simulink model "Definition_mf_2"  (R2020b)
settings: Solver=VariableStepAuto  StartTime=0.0  StopTime=8.5  RelTol=1e-3
values from neighbouring files (symbols this model uses):
  b = 0.0000313    (= 3.13e-05)    [parametre.m]
  d = 0.00000075    (= 7.5e-07)    [parametre.m]
  Ix = 0.0075    [parametre.m]
  Iy = 0.0075    [parametre.m]
  Iz = 0.013    [parametre.m]
  J = 0.00006    (= 6e-05)    [parametre.m]
  Jt = 0.0000604    (= 6.04e-05)    [parametre.m]
  k = 5.2*(10^(-3))    (= 0.0052)    [parametre.m]
  l = 0.23    [parametre.m]
  nu = 90    [parametre.m]
  r = 1/4    (= 0.25)    [parametre.m]
  to = ((R*Jt)/(k^2))    (= 1.34023668639)    [parametre.m]
libraries: pid_lib x3
settings Model: Creator=momen  LastModifiedBy=momen

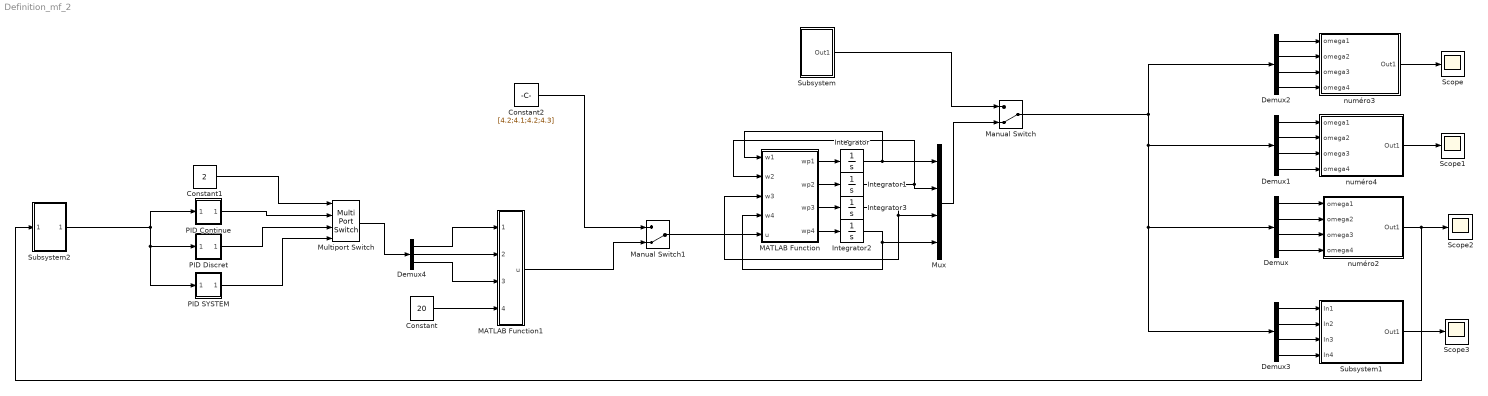
== system Definition_mf_2 ==
  Constant : Constant  Value=20
  Constant1 : Constant  Value=2
  Constant2 : Constant  Value=[4.2;4.1;4.2;4.3]
  Demux{,1..3} (4 alike) : Demux
  Demux4 : Demux  Outputs=3
  Integrator{,1..3} (4 alike) : Integrator
  MATLAB Function : MATLAB Function  TreatAsAtomicUnit=on
  MATLAB Function1 : MATLAB Function  TreatAsAtomicUnit=on
  Manual Switch : ManualSwitch  CurrentSetting=0
  Manual Switch1 : ManualSwitch  CurrentSetting=0
  Multiport Switch : MultiPortSwitch
  Mux : Mux
  PID Continue : Subsystem
  PID Discret : Subsystem
  PID SYSTEM : Subsystem
  Scope{,1..3} (4 alike) : Scope
  Subsystem : Subsystem
  Subsystem1 : Subsystem
  Subsystem2 : Subsystem
  numéro2 : Subsystem
  numéro3 : Subsystem
  numéro4 : Subsystem
  wires:
  numéro4/1(Out1) -> Scope1/1
  numéro2/1(Out1) -> Subsystem2/1(In1), Scope2/1
  Demux2/1 -> numéro3/1(omega1)
  Demux2/2 -> numéro3/2(omega2)
  Demux2/3 -> numéro3/3(omega3)
  Demux2/4 -> numéro3/4(omega4)
  Demux1/1 -> numéro4/1(omega1)
  Demux1/2 -> numéro4/2(omega2)
  Demux1/3 -> numéro4/3(omega3)
  Demux1/4 -> numéro4/4(omega4)
  Demux/4 -> numéro2/4(omega4)
  Demux/3 -> numéro2/3(omega3)
  Demux/2 -> numéro2/2(omega2)
  Demux/1 -> numéro2/1(omega1)
  Demux3/1 -> Subsystem1/1(In1)
  Demux3/2 -> Subsystem1/2(In2)
  Demux3/3 -> Subsystem1/3(In3)
  Demux3/4 -> Subsystem1/4(In4)
  Subsystem1/1(Out1) -> Scope3/1
  Constant2/1 -> Manual Switch1/1
  MATLAB Function/1(wp1) -> Integrator/1
  MATLAB Function/2(wp2) -> Integrator1/1
  MATLAB Function/3(wp3) -> Integrator3/1
  MATLAB Function/4(wp4) -> Integrator2/1
  Manual Switch/1 -> Demux3/1, Demux/1, Demux1/1, Demux2/1
  Subsystem/1(Out1) -> Manual Switch/1
  Integrator/1 -> MATLAB Function/1(w1), Mux/1
  Integrator1/1 -> Mux/2, MATLAB Function/2(w2)
  Integrator3/1 -> Mux/3, MATLAB Function/3(w3)
  Integrator2/1 -> Mux/4, MATLAB Function/4(w4)
  Mux/1 -> Manual Switch/2
  Manual Switch1/1 -> MATLAB Function/5(u)
  MATLAB Function1/1(u) -> Manual Switch1/2
  Constant/1 -> MATLAB Function1/4(v4)
  numéro3/1(Out1) -> Scope/1
  Subsystem2/1(Out1) -> PID SYSTEM/1(In1), PID Discret/1(In1), PID Continue/1(In1)
  PID Continue/1(Out1) -> Multiport Switch/2
  Demux4/1 -> MATLAB Function1/1(v1)
  Demux4/2 -> MATLAB Function1/2(v2)
  Demux4/3 -> MATLAB Function1/3(v3)
  PID Discret/1(Out1) -> Multiport Switch/3
  Multiport Switch/1 -> Demux4/1
  Constant1/1 -> Multiport Switch/1
  PID SYSTEM/1(Out1) -> Multiport Switch/4

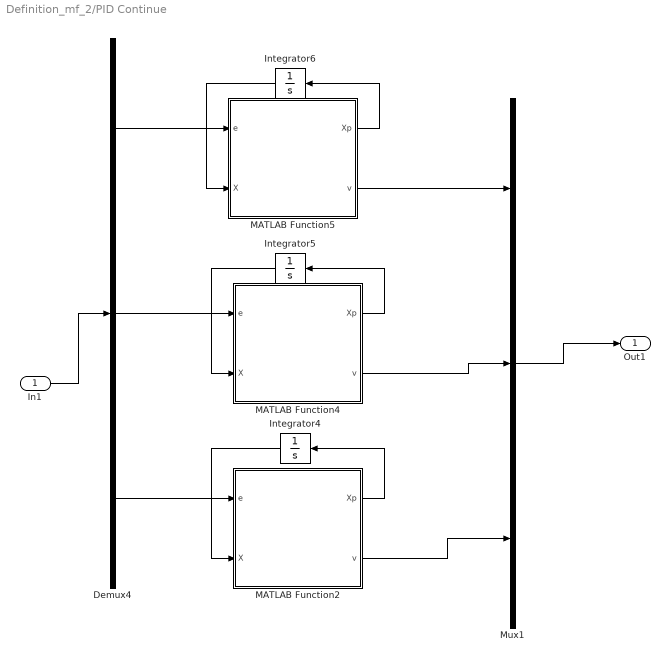
== system Definition_mf_2/PID Continue ==
  In1 : Inport
  Demux4 : Demux  Outputs=3
  Integrator4 : Integrator  InitialCondition=[0;0]
  Integrator5 : Integrator  InitialCondition=[0;0]
  Integrator6 : Integrator  InitialCondition=[0;0]
  MATLAB Function2 : MATLAB Function  TreatAsAtomicUnit=on
  MATLAB Function4 : MATLAB Function  TreatAsAtomicUnit=on
  MATLAB Function5 : MATLAB Function  TreatAsAtomicUnit=on
  Mux1 : Mux  Inputs=3
  Out1 : Outport
  wires:
  MATLAB Function5/1(Xp) -> Integrator6/1
  MATLAB Function2/1(Xp) -> Integrator4/1
  Demux4/1 -> MATLAB Function5/1(e)
  Integrator6/1 -> MATLAB Function5/2(X)
  Integrator5/1 -> MATLAB Function4/2(X)
  MATLAB Function5/2(v) -> Mux1/1
  MATLAB Function4/2(v) -> Mux1/2
  Demux4/2 -> MATLAB Function4/1(e)
  MATLAB Function4/1(Xp) -> Integrator5/1
  MATLAB Function2/2(v) -> Mux1/3
  Demux4/3 -> MATLAB Function2/1(e)
  Integrator4/1 -> MATLAB Function2/2(X)
  Mux1/1 -> Out1/1
  In1/1 -> Demux4/1

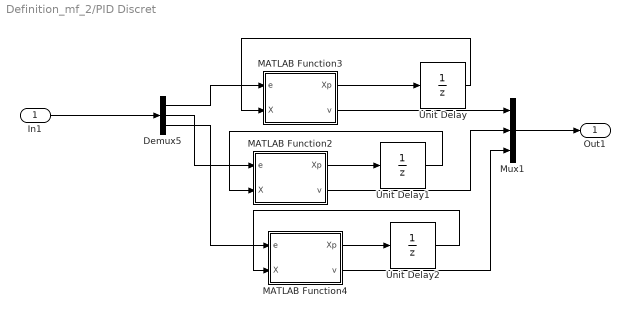
== system Definition_mf_2/PID Discret ==
  In1 : Inport
  Demux5 : Demux  Outputs=3
  MATLAB Function2 : MATLAB Function  TreatAsAtomicUnit=on
  MATLAB Function3 : MATLAB Function  TreatAsAtomicUnit=on
  MATLAB Function4 : MATLAB Function  TreatAsAtomicUnit=on
  Mux1 : Mux  Inputs=3
  Unit Delay : UnitDelay  InitialCondition=[0;0]  SampleTime=-1  HasFrameUpgradeWarning=on
  Unit Delay1 : UnitDelay  InitialCondition=[0;0]  SampleTime=-1  HasFrameUpgradeWarning=on
  Unit Delay2 : UnitDelay  InitialCondition=[0;0]  SampleTime=-1  HasFrameUpgradeWarning=on
  Out1 : Outport
  wires:
  MATLAB Function3/1(Xp) -> Unit Delay/1
  Unit Delay1/1 -> MATLAB Function2/2(X)
  MATLAB Function2/1(Xp) -> Unit Delay1/1
  Demux5/3 -> MATLAB Function4/1(e)
  MATLAB Function4/1(Xp) -> Unit Delay2/1
  MATLAB Function2/2(v) -> Mux1/2
  Unit Delay2/1 -> MATLAB Function4/2(X)
  Unit Delay/1 -> MATLAB Function3/2(X)
  Demux5/2 -> MATLAB Function2/1(e)
  MATLAB Function3/2(v) -> Mux1/1
  MATLAB Function4/2(v) -> Mux1/3
  Mux1/1 -> Out1/1
  Demux5/1 -> MATLAB Function3/1(e)
  In1/1 -> Demux5/1

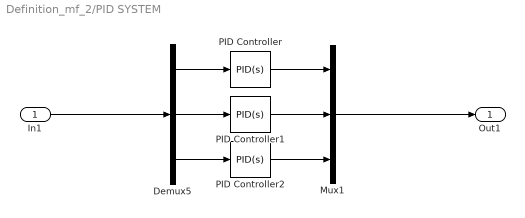
== system Definition_mf_2/PID SYSTEM ==
  In1 : Inport
  Demux5 : Demux  Outputs=3
  Mux1 : Mux  Inputs=3
  PID Controller : pid_lib/PID Controller  Controller=PID  Form=Parallel  TimeDomain=Continuous-time  UseExternalTs=off  SampleTime=-1  IntegratorMethod=Forward Euler  FilterMethod=Forward Euler  ControllerParametersSource=internal  P=0.9  I=0.3  D=0.2  UseFilter=on  N=100  TunerSelectOption=Transfer Function Based (PID Tuner App)  InitialConditionSource=internal  InitialConditionForIntegrator=0  InitialConditionForFilter=0  DifferentiatorICPrevScaledInput=0  ExternalReset=none  TrackingMode=off  Kt=1  LimitOutput=off  SatLimitsSource=internal  UpperSaturationLimit=inf  LowerSaturationLimit=-inf  LinearizeAsGain=on  AntiWindupMode=none  Kb=1  POutMin=[]  POutMax=[]  IOutMin=[]  IOutMax=[]  DOutMin=[]  DOutMax=[]  NOutMin=[]  NOutMax=[]  SumOutMin=[]  SumOutMax=[]  SaturationOutMin=[]  SaturationOutMax=[]  PParamMin=[]  PParamMax=[]  IParamMin=[]  IParamMax=[]  DParamMin=[]  DParamMax=[]  NParamMin=[]  NParamMax=[]  KbParamMin=[]  KbParamMax=[]  KtParamMin=[]  KtParamMax=[]  KbOutMin=[]  KbOutMax=[]  KtOutMin=[]  KtOutMax=[]  IntegratorOutMin=[]  IntegratorOutMax=[]  FilterOutMin=[]  FilterOutMax=[]  SumI1OutMin=[]  SumI1OutMax=[]  SumI2OutMin=[]  SumI2OutMax=[]  SumI3OutMin=[]  SumI3OutMax=[]  SumI4OutMin=[]  SumI4OutMax=[]  SumDOutMin=[]  SumDOutMax=[]  DifferentiatorOutMin=[]  DifferentiatorOutMax=[]  FilterDiffOutCoefMin=[]  FilterDiffOutCoefMax=[]  ReciprocalOutMin=[]  ReciprocalOutMax=[]  SumDenOutMin=[]  SumDenOutMax=[]  SumNumOutMin=[]  SumNumOutMax=[]  DivideOutMin=[]  DivideOutMax=[]  UdiffTsProdOutMin=[]  UdiffTsProdOutMax=[]  NTsProdOutMin=[]  NTsProdOutMax=[]  UintegralTsProdOutMin=[]  UintegralTsProdOutMax=[]  UngainTsProdOutMin=[]  UngainTsProdOutMax=[]  IntegratorContinuousStateAttributes=''  IntegratorStateMustResolveToSignalObject=off  IntegratorRTWStateStorageClass=Auto  FilterContinuousStateAttributes=''  FilterStateMustResolveToSignalObject=off  FilterRTWStateStorageClass=Auto  ParallelPVariant=InternalParameters  IdealPVariant=Disabled  IVariant=InternalParameters  DVariant=InternalParameters  IntegratorVariant=Continuous  SatVariant=Disabled  AWVariant=Passthrough  PCopyVariant=Disabled  TRVariant=Disabled  FdbkBlocksVariant=Forward  IdealPFdbkVariant=Disabled  SatFdbkVariant=Disabled  DerivativeFilterVariant=ContFilter  NVariant=InternalParameters  NCopyVariant=Disabled  FilterICVariant=InternalICsFilter  IntegratorICVariant=InternalICs  ExternalResetVariant=Disabled  TRSumVariant=Passthrough  SumFdbkVariant=Disabled  SumVariant=Sum_PID  TsampFilterVariant=InternalTs  TsampNgainVariant=Passthrough  TsampIntegralVariant=Passthrough  ExternalSaturationOutDataTypeStr=Inherit: Same as second input
  PID Controller1 : pid_lib/PID Controller  Controller=PID  Form=Parallel  TimeDomain=Continuous-time  UseExternalTs=off  SampleTime=-1  IntegratorMethod=Forward Euler  FilterMethod=Forward Euler  ControllerParametersSource=internal  P=0.9  I=0.3  D=0.2  UseFilter=on  N=100  TunerSelectOption=Transfer Function Based (PID Tuner App)  InitialConditionSource=internal  InitialConditionForIntegrator=0  InitialConditionForFilter=0  DifferentiatorICPrevScaledInput=0  ExternalReset=none  TrackingMode=off  Kt=1  LimitOutput=off  SatLimitsSource=internal  UpperSaturationLimit=inf  LowerSaturationLimit=-inf  LinearizeAsGain=on  AntiWindupMode=none  Kb=1  POutMin=[]  POutMax=[]  IOutMin=[]  IOutMax=[]  DOutMin=[]  DOutMax=[]  NOutMin=[]  NOutMax=[]  SumOutMin=[]  SumOutMax=[]  SaturationOutMin=[]  SaturationOutMax=[]  PParamMin=[]  PParamMax=[]  IParamMin=[]  IParamMax=[]  DParamMin=[]  DParamMax=[]  NParamMin=[]  NParamMax=[]  KbParamMin=[]  KbParamMax=[]  KtParamMin=[]  KtParamMax=[]  KbOutMin=[]  KbOutMax=[]  KtOutMin=[]  KtOutMax=[]  IntegratorOutMin=[]  IntegratorOutMax=[]  FilterOutMin=[]  FilterOutMax=[]  SumI1OutMin=[]  SumI1OutMax=[]  SumI2OutMin=[]  SumI2OutMax=[]  SumI3OutMin=[]  SumI3OutMax=[]  SumI4OutMin=[]  SumI4OutMax=[]  SumDOutMin=[]  SumDOutMax=[]  DifferentiatorOutMin=[]  DifferentiatorOutMax=[]  FilterDiffOutCoefMin=[]  FilterDiffOutCoefMax=[]  ReciprocalOutMin=[]  ReciprocalOutMax=[]  SumDenOutMin=[]  SumDenOutMax=[]  SumNumOutMin=[]  SumNumOutMax=[]  DivideOutMin=[]  DivideOutMax=[]  UdiffTsProdOutMin=[]  UdiffTsProdOutMax=[]  NTsProdOutMin=[]  NTsProdOutMax=[]  UintegralTsProdOutMin=[]  UintegralTsProdOutMax=[]  UngainTsProdOutMin=[]  UngainTsProdOutMax=[]  IntegratorContinuousStateAttributes=''  IntegratorStateMustResolveToSignalObject=off  IntegratorRTWStateStorageClass=Auto  FilterContinuousStateAttributes=''  FilterStateMustResolveToSignalObject=off  FilterRTWStateStorageClass=Auto  ParallelPVariant=InternalParameters  IdealPVariant=Disabled  IVariant=InternalParameters  DVariant=InternalParameters  IntegratorVariant=Continuous  SatVariant=Disabled  AWVariant=Passthrough  PCopyVariant=Disabled  TRVariant=Disabled  FdbkBlocksVariant=Forward  IdealPFdbkVariant=Disabled  SatFdbkVariant=Disabled  DerivativeFilterVariant=ContFilter  NVariant=InternalParameters  NCopyVariant=Disabled  FilterICVariant=InternalICsFilter  IntegratorICVariant=InternalICs  ExternalResetVariant=Disabled  TRSumVariant=Passthrough  SumFdbkVariant=Disabled  SumVariant=Sum_PID  TsampFilterVariant=InternalTs  TsampNgainVariant=Passthrough  TsampIntegralVariant=Passthrough  ExternalSaturationOutDataTypeStr=Inherit: Same as second input
  PID Controller2 : pid_lib/PID Controller  Controller=PID  Form=Parallel  TimeDomain=Continuous-time  UseExternalTs=off  SampleTime=-1  IntegratorMethod=Forward Euler  FilterMethod=Forward Euler  ControllerParametersSource=internal  P=0.06  I=0.3  D=0.02  UseFilter=on  N=100  TunerSelectOption=Transfer Function Based (PID Tuner App)  InitialConditionSource=internal  InitialConditionForIntegrator=0  InitialConditionForFilter=0  DifferentiatorICPrevScaledInput=0  ExternalReset=none  TrackingMode=off  Kt=1  LimitOutput=off  SatLimitsSource=internal  UpperSaturationLimit=inf  LowerSaturationLimit=-inf  LinearizeAsGain=on  AntiWindupMode=none  Kb=1  POutMin=[]  POutMax=[]  IOutMin=[]  IOutMax=[]  DOutMin=[]  DOutMax=[]  NOutMin=[]  NOutMax=[]  SumOutMin=[]  SumOutMax=[]  SaturationOutMin=[]  SaturationOutMax=[]  PParamMin=[]  PParamMax=[]  IParamMin=[]  IParamMax=[]  DParamMin=[]  DParamMax=[]  NParamMin=[]  NParamMax=[]  KbParamMin=[]  KbParamMax=[]  KtParamMin=[]  KtParamMax=[]  KbOutMin=[]  KbOutMax=[]  KtOutMin=[]  KtOutMax=[]  IntegratorOutMin=[]  IntegratorOutMax=[]  FilterOutMin=[]  FilterOutMax=[]  SumI1OutMin=[]  SumI1OutMax=[]  SumI2OutMin=[]  SumI2OutMax=[]  SumI3OutMin=[]  SumI3OutMax=[]  SumI4OutMin=[]  SumI4OutMax=[]  SumDOutMin=[]  SumDOutMax=[]  DifferentiatorOutMin=[]  DifferentiatorOutMax=[]  FilterDiffOutCoefMin=[]  FilterDiffOutCoefMax=[]  ReciprocalOutMin=[]  ReciprocalOutMax=[]  SumDenOutMin=[]  SumDenOutMax=[]  SumNumOutMin=[]  SumNumOutMax=[]  DivideOutMin=[]  DivideOutMax=[]  UdiffTsProdOutMin=[]  UdiffTsProdOutMax=[]  NTsProdOutMin=[]  NTsProdOutMax=[]  UintegralTsProdOutMin=[]  UintegralTsProdOutMax=[]  UngainTsProdOutMin=[]  UngainTsProdOutMax=[]  IntegratorContinuousStateAttributes=''  IntegratorStateMustResolveToSignalObject=off  IntegratorRTWStateStorageClass=Auto  FilterContinuousStateAttributes=''  FilterStateMustResolveToSignalObject=off  FilterRTWStateStorageClass=Auto  ParallelPVariant=InternalParameters  IdealPVariant=Disabled  IVariant=InternalParameters  DVariant=InternalParameters  IntegratorVariant=Continuous  SatVariant=Disabled  AWVariant=Passthrough  PCopyVariant=Disabled  TRVariant=Disabled  FdbkBlocksVariant=Forward  IdealPFdbkVariant=Disabled  SatFdbkVariant=Disabled  DerivativeFilterVariant=ContFilter  NVariant=InternalParameters  NCopyVariant=Disabled  FilterICVariant=InternalICsFilter  IntegratorICVariant=InternalICs  ExternalResetVariant=Disabled  TRSumVariant=Passthrough  SumFdbkVariant=Disabled  SumVariant=Sum_PID  TsampFilterVariant=InternalTs  TsampNgainVariant=Passthrough  TsampIntegralVariant=Passthrough  ExternalSaturationOutDataTypeStr=Inherit: Same as second input
  Out1 : Outport
  wires:
  In1/1 -> Demux5/1
  Demux5/3 -> PID Controller2/1
  Demux5/1 -> PID Controller/1
  Demux5/2 -> PID Controller1/1
  Mux1/1 -> Out1/1
  PID Controller/1 -> Mux1/1
  PID Controller1/1 -> Mux1/2
  PID Controller2/1 -> Mux1/3

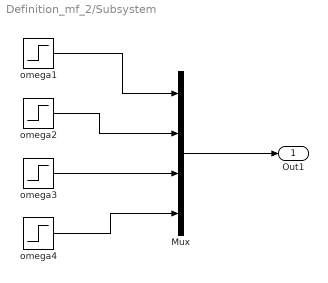
== system Definition_mf_2/Subsystem ==
  Mux : Mux
  omega{1..4} (4 alike) : Step  Time=2  After=150  SampleTime=0
  Out1 : Outport
  wires:
  omega3/1 -> Mux/3
  omega2/1 -> Mux/2
  omega1/1 -> Mux/1
  omega4/1 -> Mux/4
  Mux/1 -> Out1/1

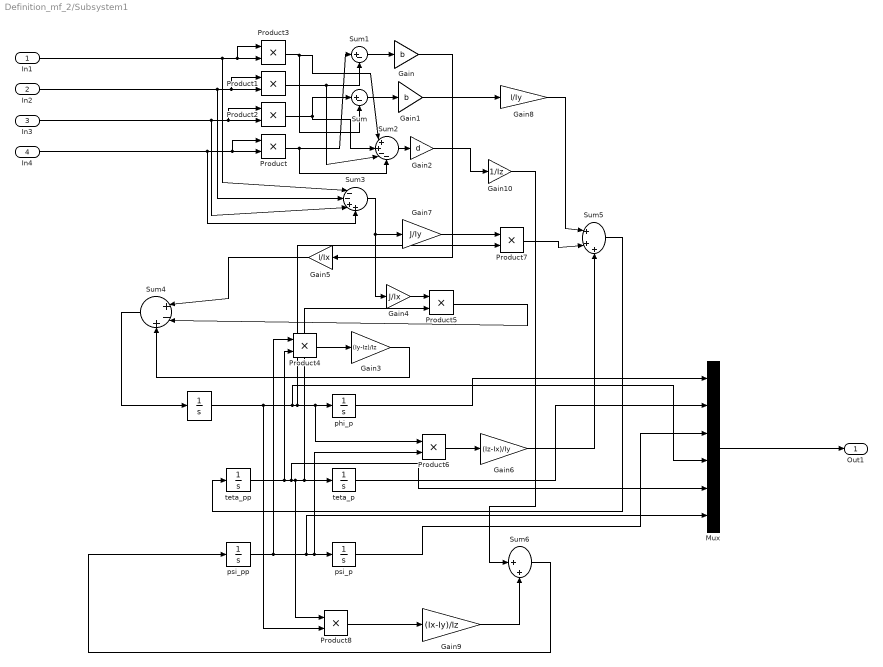
== system Definition_mf_2/Subsystem1 ==
  In1 : Inport
  In2 : Inport  Port=2
  In3 : Inport  Port=3
  In4 : Inport  Port=4
  " " : Integrator
  Gain : Gain  Gain=b
  Gain1 : Gain  Gain=b
  Gain10 : Gain  Gain=1/Iz
  Gain2 : Gain  Gain=d
  Gain3 : Gain  Gain=(Iy-Iz)/Iz
  Gain4 : Gain  Gain=J/Ix
  Gain5 : Gain  Gain=l/Ix
  Gain6 : Gain  Gain=(Iz-Ix)/Iy
  Gain7 : Gain  Gain=J/Iy
  Gain8 : Gain  Gain=l/Iy
  Gain9 : Gain  Gain=(Ix-Iy)/Iz
  Mux : Mux  Inputs=6
  Product{,1..8} (9 alike) : Product
  Sum : Sum  Inputs=|+-
  Sum1 : Sum  Inputs=|+-
  Sum2 : Sum  Inputs=|++--
  Sum3 : Sum  Inputs=|--++
  Sum4 : Sum  Inputs=|+-+
  Sum5 : Sum  Inputs=|+++
  Sum6 : Sum  Inputs=|++
  phi_p : Integrator
  psi_p : Integrator
  psi_pp : Integrator
  teta_p : Integrator
  teta_pp : Integrator
  Out1 : Outport
  wires:
  In2/1 -> Sum3/2, Product1/1, Product1/2
  Product8/1 -> Gain9/1
  Product5/1 -> Sum4/2
  Product2/1 -> Sum2/2, Sum/1
  Product1/1 -> Sum2/3, Sum1/2
  Product4/1 -> Gain3/1
  " "/1 -> Product8/2, Mux/4, Product7/2, Product6/1, phi_p/1
  Sum2/1 -> Gain2/1
  Product6/1 -> Gain6/1
  Gain6/1 -> Sum5/3
  In4/1 -> Sum3/4, Product/1, Product/2
  Sum1/1 -> Gain/1
  In1/1 -> Product3/2, Product3/1, Sum3/1
  teta_pp/1 -> Product4/2, Mux/5, Product8/1, teta_p/1, Product5/2
  Gain10/1 -> Sum6/1
  Sum3/1 -> Gain4/1, Gain7/1
  Product3/1 -> Sum2/1, Sum/2
  Gain8/1 -> Sum5/1
  psi_pp/1 -> Product4/1, Mux/6, Product6/2, psi_p/1
  Product/1 -> Sum2/4, Sum1/1
  Gain1/1 -> Gain8/1
  Gain9/1 -> Sum6/2
  Sum/1 -> Gain1/1
  Sum5/1 -> teta_pp/1
  Gain3/1 -> Sum4/3
  In3/1 -> Sum3/3, Product2/1, Product2/2
  Gain/1 -> Gain5/1
  Gain7/1 -> Product7/1
  Gain4/1 -> Product5/1
  Sum6/1 -> psi_pp/1
  teta_p/1 -> Mux/2
  phi_p/1 -> Mux/1
  Gain5/1 -> Sum4/1
  Sum4/1 -> " "/1
  Product7/1 -> Sum5/2
  psi_p/1 -> Mux/3
  Gain2/1 -> Gain10/1
  Mux/1 -> Out1/1

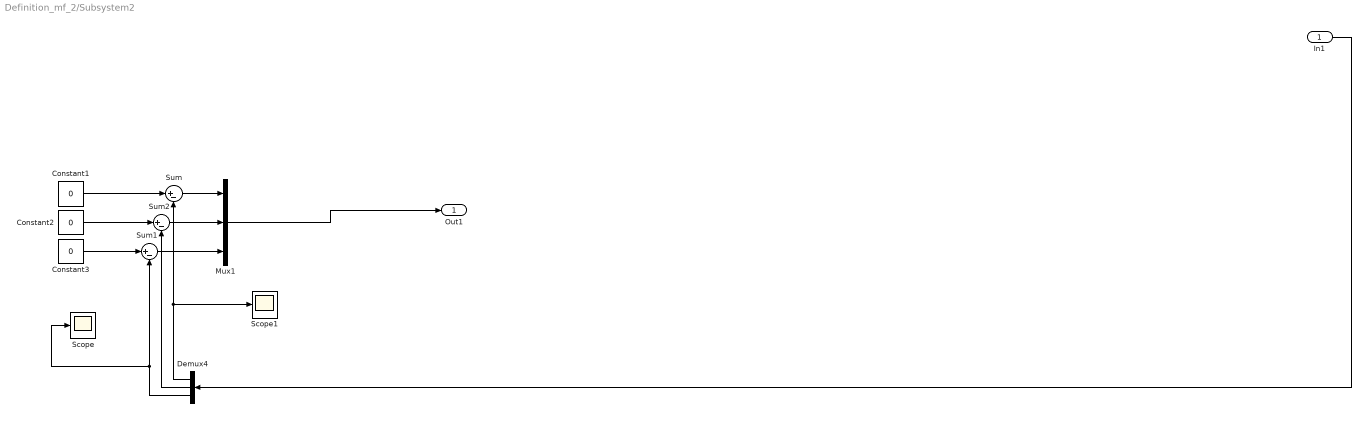
== system Definition_mf_2/Subsystem2 ==
  In1 : Inport
  Constant1 : Constant  Value=0
  Constant2 : Constant  Value=0
  Constant3 : Constant  Value=0
  Demux4 : Demux  Outputs=3
  Mux1 : Mux  Inputs=3
  Scope : Scope
  Scope1 : Scope
  Sum : Sum  Inputs=|+-
  Sum1 : Sum  Inputs=|+-
  Sum2 : Sum  Inputs=|+-
  Out1 : Outport
  wires:
  Demux4/1 -> Sum/2, Scope1/1
  Demux4/3 -> Scope/1, Sum1/2
  Sum1/1 -> Mux1/3
  Constant3/1 -> Sum1/1
  Demux4/2 -> Sum2/2
  Sum/1 -> Mux1/1
  Constant2/1 -> Sum2/1
  Constant1/1 -> Sum/1
  Sum2/1 -> Mux1/2
  Mux1/1 -> Out1/1
  In1/1 -> Demux4/1

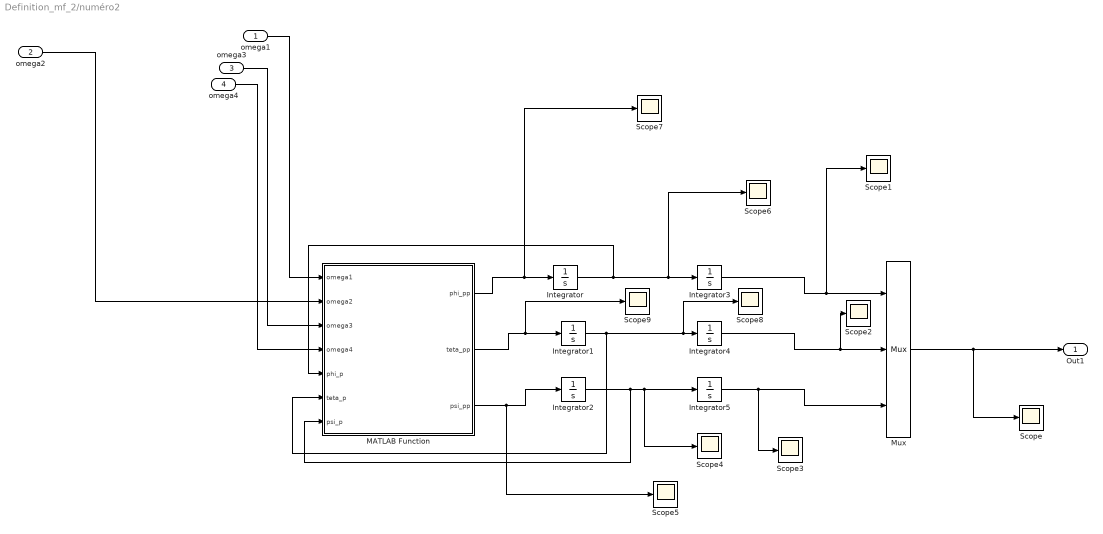
== system Definition_mf_2/numéro2 ==
  omega1 : Inport
  omega2 : Inport  Port=2
  omega3 : Inport  Port=3
  omega4 : Inport  Port=4
  Integrator : Integrator
  Integrator1 : Integrator
  Integrator2 : Integrator
  Integrator3 : Integrator  InitialCondition=pi/4
  Integrator4 : Integrator  InitialCondition=pi/4
  Integrator5 : Integrator  InitialCondition=pi/4
  MATLAB Function : MATLAB Function  TreatAsAtomicUnit=on
  Mux : Mux  Inputs=3
  Scope{,1..9} (10 alike) : Scope
  Out1 : Outport
  wires:
  Integrator3/1 -> Scope1/1, Mux/1
  MATLAB Function/2(teta_pp) -> Scope9/1, Integrator1/1
  Integrator1/1 -> MATLAB Function/6(teta_p), Scope8/1, Integrator4/1
  Integrator/1 -> MATLAB Function/5(phi_p), Scope6/1, Integrator3/1
  omega2/1 -> MATLAB Function/2(omega2)
  Integrator2/1 -> MATLAB Function/7(psi_p), Scope4/1, Integrator5/1
  Integrator4/1 -> Scope2/1, Mux/2
  MATLAB Function/1(phi_pp) -> Scope7/1, Integrator/1
  MATLAB Function/3(psi_pp) -> Scope5/1, Integrator2/1
  omega4/1 -> MATLAB Function/4(omega4)
  omega3/1 -> MATLAB Function/3(omega3)
  omega1/1 -> MATLAB Function/1(omega1)
  Mux/1 -> Scope/1, Out1/1
  Integrator5/1 -> Scope3/1, Mux/3

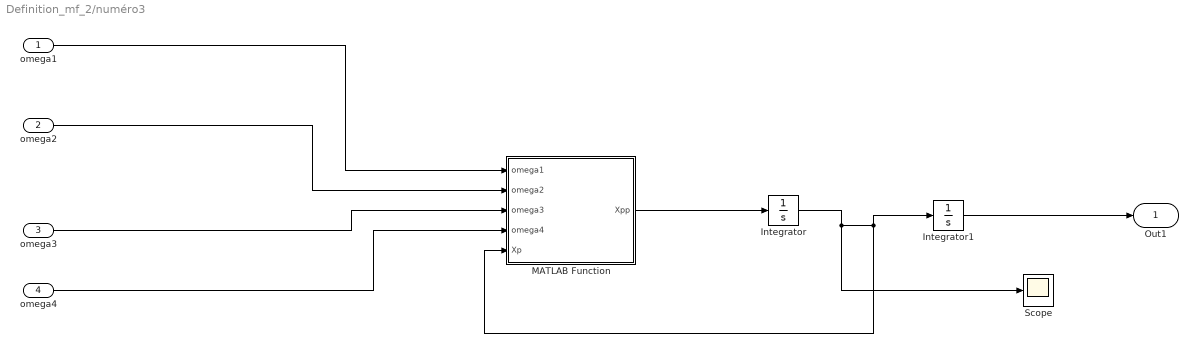
== system Definition_mf_2/numéro3 ==
  omega1 : Inport
  omega2 : Inport  Port=2
  omega3 : Inport  Port=3
  omega4 : Inport  Port=4
  Integrator : Integrator  InitialCondition=[0;0;0]
  Integrator1 : Integrator  InitialCondition=[0;0;0]
  MATLAB Function : MATLAB Function  TreatAsAtomicUnit=on
  Scope : Scope
  Out1 : Outport
  wires:
  MATLAB Function/1(Xpp) -> Integrator/1
  omega1/1 -> MATLAB Function/1(omega1)
  omega3/1 -> MATLAB Function/3(omega3)
  omega2/1 -> MATLAB Function/2(omega2)
  Integrator1/1 -> Out1/1
  omega4/1 -> MATLAB Function/4(omega4)
  Integrator/1 -> Scope/1, Integrator1/1, MATLAB Function/5(Xp)

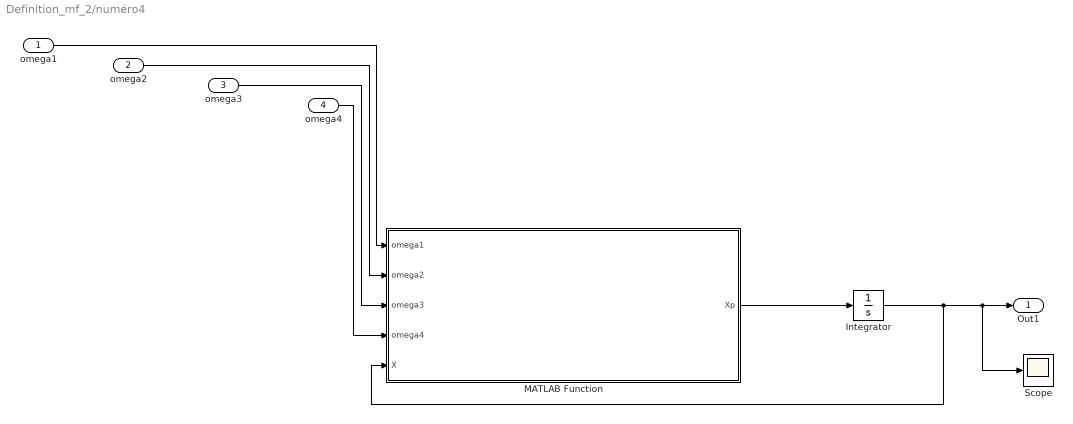
== system Definition_mf_2/numéro4 ==
  omega1 : Inport
  omega2 : Inport  Port=2
  omega3 : Inport  Port=3
  omega4 : Inport  Port=4
  Integrator : Integrator  InitialCondition=[0.785;0.785;0.785;0;0;0]
  MATLAB Function : MATLAB Function  TreatAsAtomicUnit=on
  Scope : Scope
  Out1 : Outport
  wires:
  Integrator/1 -> Scope/1, Out1/1, MATLAB Function/5(X)
  omega4/1 -> MATLAB Function/4(omega4)
  omega1/1 -> MATLAB Function/1(omega1)
  MATLAB Function/1(Xp) -> Integrator/1
  omega3/1 -> MATLAB Function/3(omega3)
  omega2/1 -> MATLAB Function/2(omega2)

== matlab function Definition_mf_2/MATLAB Function1 ==
  data: v1 input; u output; v2 input; v3 input; v4 input
function u = T(v1,v2,v3,v4)
u=[0;0;0;0];
u(1)=(-0.5*v2 -0.25*v3 + 0.25*v4 );
u(2)=(-0.5*v1 +0.25*v3 + 0.25*v4 );
u(3)=( 0.5*v2 -0.25*v3 + 0.25*v4 );
u(4)=( 0.5*v1 +0.25*v3 + 0.25*v4 );

== matlab function Definition_mf_2/PID Continue/MATLAB Function2 ==
  data: e input; Xp output; X input; v output
function [Xp,v]= fcn(e,X)
Kp=0.8
Ki=0
Kd=0.5
N= 100
Xp=[0;0];
Xp(1) = e;
Xp(2) = N*(Kd*e-X(2));
Xp=[Xp(1);Xp(2)];
v = Kp*e+Ki*X(1)+Xp(2);

== matlab function Definition_mf_2/PID Discret/MATLAB Function3 ==
  data: e input; Xp output; X input; v output; Te parameter
function [Xp,v]= fcn(e,X,Te)
Kp=0.8
Ki=0
Kd=0.4
N= 100
Xp=[0;0];
Xp(1) = X(1) + Te*e;
Xp(2) = X(2) +Te*N*(Kd*e-X(2));
Xp=[Xp(1);Xp(2)];
v = Kp*e+Ki*X(1)+N*(Kd*e-X(2));

== matlab function Definition_mf_2/PID Continue/MATLAB Function4 ==
  data: e input; Xp output; X input; v output
function [Xp,v]= fcn(e,X)
Kp=0.8
Ki=0
Kd=0.5
N= 100
Xp=[0;0];
Xp(1) = e;
Xp(2) = N*(Kd*e-X(2));
Xp=[Xp(1);Xp(2)];
v = Kp*e+Ki*X(1)+Xp(2);

== matlab function Definition_mf_2/PID Continue/MATLAB Function5 ==
  data: e input; Xp output; X input; v output
function [Xp,v]= fcn(e,X)
Kp=0.8
Ki=0
Kd=0.5
N= 100
Xp=[0;0];
Xp(1) = e;
Xp(2) = N*(Kd*e-X(2));
Xp=[Xp(1);Xp(2)];
v = Kp*e+Ki*X(1)+Xp(2);

== matlab function Definition_mf_2/PID Discret/MATLAB Function2 ==
  data: e input; Xp output; X input; v output; Te parameter
function [Xp,v]= fcn(e,X,Te)
Kp=0.8
Ki=0
Kd=0.4
N= 100
Xp=[0;0];
Xp(1) = X(1) + Te*e;
Xp(2) = X(2) +Te*N*(Kd*e-X(2));
Xp=[Xp(1);Xp(2)];
v = Kp*e+Ki*X(1)+N*(Kd*e-X(2));

== matlab function Definition_mf_2/PID Discret/MATLAB Function4 ==
  data: e input; Xp output; X input; v output; Te parameter
function [Xp,v]= fcn(e,X,Te)
Kp=0.8
Ki=0
Kd=0.5
N= 100
Xp=[0;0];
Xp(1) = X(1) + Te*e;
Xp(2) = X(2) +Te*N*(Kd*e-X(2));
Xp=[Xp(1);Xp(2)];
v = Kp*e+Ki*X(1)+N*(Kd*e-X(2));

== matlab function Definition_mf_2/numéro4/MATLAB Function ==
  data: omega1 input; Xp output; omega2 input; omega3 input; omega4 input; X input; Ix parameter; Iy parameter; Iz parameter; J parameter; b parameter; d parameter; l parameter
function Xp = n4(omega1,omega2,omega3,omega4,X,Ix, Iy, Iz, J, b, d, l)
Xp = [0;0;0;0;0;0];
U1 = 0;
U2 = 0;
U3 = 0;
omega =0;
U1 = b*((omega4^2)-(omega2^2));
U2 = b*(omega3^2-omega1^2);
U3 = d*(-omega1^2-omega3^2+omega2^2+omega4^2);
omega = omega2+omega4-omega1-omega3;
Xp(1) = X(4);
Xp(2) = X(5);
Xp(3) = X(6);
Xp(4) = X(5)*X(6)*((Iy-Iz)/Ix)-(J/Ix)*X(5)*omega +(l/Ix)*U1;
Xp(5) = X(4)*X(6)*((Iz-Ix)/Iy)+(J/Iy)*X(4)*omega +(l/Ix)*U2;
Xp(6) = X(4)*X(5)*((Ix-Iy)/Iz)+(1/Iz)*U3;
Xp = [Xp(1);Xp(2);Xp(3);Xp(4);Xp(5);Xp(6)];

== matlab function Definition_mf_2/numéro3/MATLAB Function ==
  data: omega1 input; Xpp output; omega2 input; omega3 input; omega4 input; Xp input; Ix parameter; Iy parameter; Iz parameter; J parameter; b parameter; d parameter; l parameter
function Xpp = n3(omega1,omega2,omega3,omega4,Xp,Ix, Iy, Iz, J,b, d,l)
Xpp = [0; 0; 0];
U1 = 0;
U2 = 0;
U3 = 0;
omega = 0;
U1 = b*((omega4^2)-(omega2^2));
U2 = b*(omega3^2-omega1^2);
U3 = d*(omega1^2+omega3^2-omega2^2-omega4^2);
omega = omega2+omega4-omega1-omega3;
Xpp(1) = Xp(2)*Xp(3)*((Iy-Iz)/Ix)-(J/Ix)*Xp(2)*omega +(l/Ix)*U1;
Xpp(2) = Xp(1)*Xp(3)*((Iz-Ix)/Iy)+(J/Iy)*Xp(1)*omega +(l/Ix)*U2;
Xpp(3) = Xp(1)*Xp(2)*((Ix-Iy)/Iz)+(1/Iz)*U3;
Xpp = [Xpp(1); Xpp(2);Xpp(3)];

== matlab function Definition_mf_2/numéro2/MATLAB Function ==
  data: omega1 input; phi_pp output; omega2 input; omega3 input; omega4 input; phi_p input; teta_p input; psi_p input; Ix parameter; Iy parameter; Iz parameter; J parameter; b parameter; d parameter; l parameter; teta_pp output; psi_pp output
function [phi_pp,teta_pp,psi_pp]= fcn(omega1,omega2,omega3,omega4,phi_p,teta_p,psi_p,Ix, Iy, Iz, J, b, d, l)
phi_pp = 0;
teta_pp = 0;
psi_pp = 0;
U1 = 0;
U2 = 0;
U3 = 0;
omega =0;
U1 = b*((omega4^2)-(omega2^2));
U2 = b*(omega3^2-omega1^2);
U3 = d*(-omega1^2-omega3^2+omega2^2+omega4^2);
omega = omega2+omega4-omega1-omega3;
phi_pp = teta_p*psi_p*((Iy-Iz)/Ix)-(J/Ix)*teta_p*omega +(l/Ix)*U1;
teta_pp = phi_p*psi_p*((Iz-Ix)/Iy)+(J/Iy)*phi_p*omega +(l/Ix)*U2;
psi_pp =phi_p*teta_p*((Ix-Iy)/Iz)+(1/Iz)*U3;

== matlab function Definition_mf_2/MATLAB Function ==
  data: w1 input; w2 input; w3 input; w4 input; u input; wp1 output; wp2 output; wp3 output; wp4 output; to parameter; nu parameter; r parameter; Jt parameter; k parameter; d parameter
function [wp1,wp2,wp3,wp4]= fcn(w1,w2,w3,w4,u,to, nu, r, Jt, k,d)
wp1 = 0;
wp2 = 0;
wp3 = 0;
wp4 = 0;
wp1 = -(1/to)*w1-(d/(nu*(r^3)*Jt))*(w1^2)+(u(1)/(k*to));
wp2 = -(1/to)*w2-(d/(nu*(r^3)*Jt))*(w2^2)+(u(2)/(k*to));
wp3 = -(1/to)*w3-(d/(nu*(r^3)*Jt))*(w3^2)+(u(3)/(k*to));
wp4 = -(1/to)*w4-(d/(nu*(r^3)*Jt))*(w4^2)+(u(4)/(k*to));
